simulink model "retail_store"  (R2014a)
settings: Solver=ode3  SolverMode=SingleTasking  StartTime=0.0  StopTime=24*3600  FixedStep=1  RelTol=1e-3
libraries: refrigeration x8
settings Model: Creator=avenger  LastModifiedBy=avenger
settings SolverCC: AutoInsertRateTranBlk=on
settings DataIOCC: LimitDataPoints=off
settings OptimizationCC: SimCompilerOptimization=off
settings DebuggingCC: MergeDetectMultiDrivingBlocksExec=error  FrameProcessingCompatibilityMsg=error
settings RTWCC: RTWCompilerOptimization=off

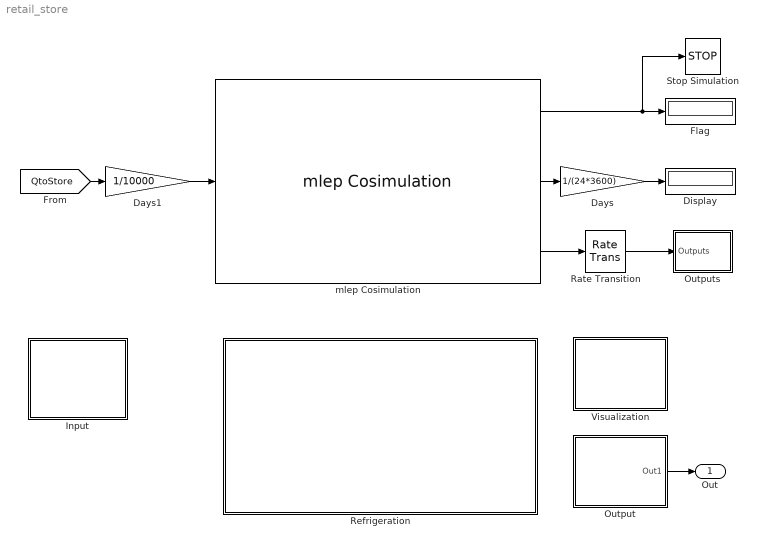
== system retail_store ==
  Days : Gain  Gain=1/(24*3600)
  Days1 : Gain  Gain=1/10000
  Display : Display
  Flag : Display
  Input : Subsystem
  Output : Subsystem
  Outputs : Subsystem
  Rate Transition : RateTransition
  Refrigeration : Subsystem
  Stop Simulation : Stop
  Visualization : Subsystem
  mlep Cosimulation : refrigeration/mlep Cosimulation  progname='runenergyplus'  idf='retail_810_cosim'  weather='USA_IL_Chicago-OHare.Intl.AP.725300_TMY3'  timeout=10000  step=300  numinput=1  numoutput=5  bcvtbpath='/home/ubuntu/mlep/bcvtb'
  Out : Outport  InitialOutput=0
  wires:
  mlep Cosimulation/2 -> Days/1
  mlep Cosimulation/1 -> Stop Simulation/1, Flag/1
  Days/1 -> Display/1
  mlep Cosimulation/3 -> Rate Transition/1
  [QtoStore] -> Days1/1
  Rate Transition/1 -> Outputs/1(Outputs)
  Days1/1 -> mlep Cosimulation/1
  Output/1(Out1) -> Out/1

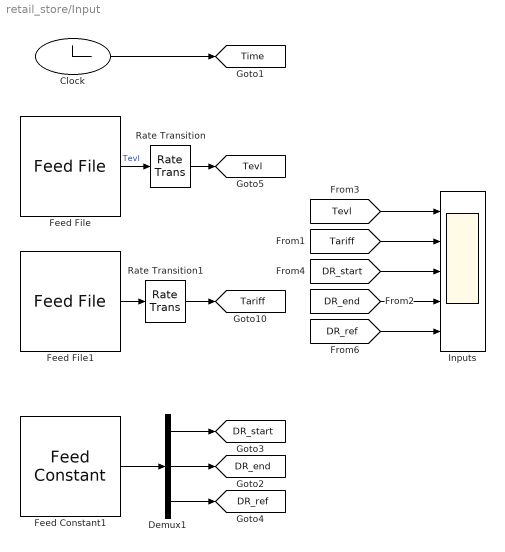
== system retail_store/Input ==
  Clock : Clock
  Demux1 : Demux  Outputs=3
  Feed Constant1 : refrigeration/Utilities/Feed Constant  filename='constant.txt'  timestep=300  numinput=3
  Feed File : refrigeration/Utilities/Feed File  filename='input.txt'  timestep=300  feedstep=3600
  Feed File1 : refrigeration/Utilities/Feed File  filename='input.txt'  timestep=300  feedstep=3600
  Inputs : Scope  NumInputPorts=5
      settings: ShowLegends=on  TimeRange=90000  YMin=0~0.02~14~14~399999  YMax=25~0.1~16~16~400001  SaveName=ScopeData3  SampleInput=on
  Rate Transition : RateTransition
  Rate Transition1 : RateTransition
  tag scope: DR_end=global, DR_ref=global, DR_start=global, Tariff=global, Tevl=global, Time=global
  wires:
  Feed File/1 -> Rate Transition/1  "Tevl"
  Clock/1 -> [Time]
  Feed File1/1 -> Rate Transition1/1
  Feed Constant1/1 -> Demux1/1
  [Tevl] -> Inputs/1
  [Tariff] -> Inputs/2
  Demux1/1 -> [DR_start]
  Demux1/2 -> [DR_end]
  Demux1/3 -> [DR_ref]
  [DR_start] -> Inputs/3
  [DR_end] -> Inputs/4
  [DR_ref] -> Inputs/5
  Rate Transition/1 -> [Tevl]
  Rate Transition1/1 -> [Tariff]

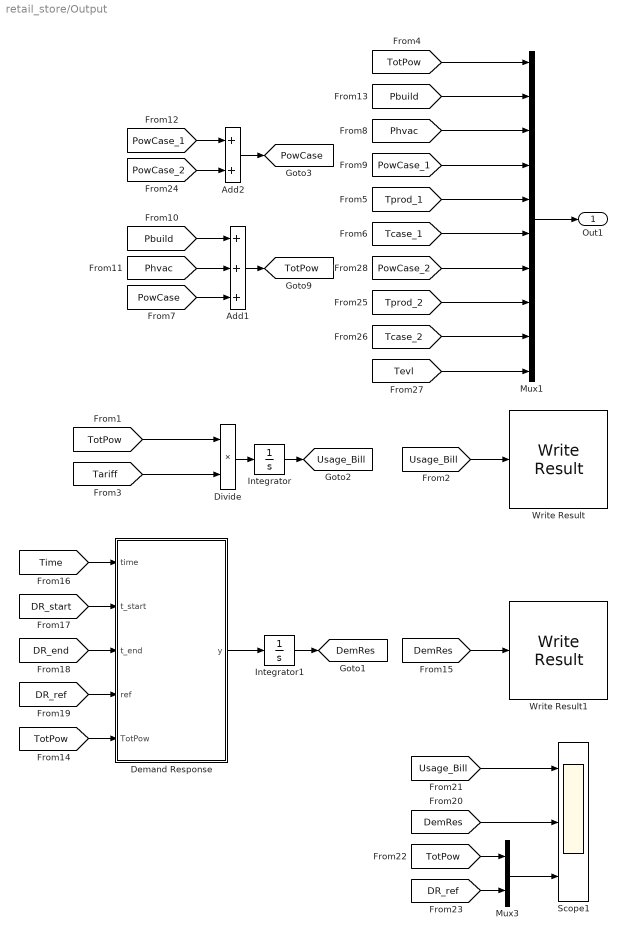
== system retail_store/Output ==
  Add1 : Sum  Inputs=+++
  Add2 : Sum
  Demand Response : MATLAB Function  TreatAsAtomicUnit=on
  Divide : Product  Inputs=**
  Integrator : Integrator  UpperSaturationLimit=10^7  LowerSaturationLimit=-10^7
  Integrator1 : Integrator  UpperSaturationLimit=10^7  LowerSaturationLimit=-10^7
  Mux1 : Mux  Inputs=10
  Mux3 : Mux  Inputs=2
  Scope1 : Scope  NumInputPorts=3
      settings: ShowLegends=on  TimeRange=90000  YMin=-200000000~0~-100000  YMax=1200000000~1200000000~500000  SaveName=ScopeData5
  Write Result : refrigeration/Utilities/Write Result  filename='result1.txt'  timestep=3600
  Write Result1 : refrigeration/Utilities/Write Result  filename='result2.txt'  timestep=3600
  Out1 : Outport  InitialOutput=0
  tag scope: DemRes=global, PowCase=global, TotPow=global, Usage_Bill=global
  wires:
  [Tariff] -> Divide/2
  Divide/1 -> Integrator/1
  [Pbuild] -> Add1/1
  [Phvac] -> Add1/2
  Add1/1 -> [TotPow]
  [Pbuild] -> Mux1/2
  [Tcase_1] -> Mux1/6
  [Tprod_1] -> Mux1/5
  [Phvac] -> Mux1/3
  [PowCase_1] -> Mux1/4
  [TotPow] -> Mux1/1
  Mux1/1 -> Out1/1
  Integrator/1 -> [Usage_Bill]
  [Usage_Bill] -> Write Result/1
  [DemRes] -> Write Result1/1
  [Time] -> Demand Response/1(time)
  [DR_start] -> Demand Response/2(t_start)
  [DR_end] -> Demand Response/3(t_end)
  [DR_ref] -> Demand Response/4(ref)
  [TotPow] -> Demand Response/5(TotPow)
  Demand Response/1(y) -> Integrator1/1
  Integrator1/1 -> [DemRes]
  [DemRes] -> Scope1/2
  [Usage_Bill] -> Scope1/1
  Mux3/1 -> Scope1/3
  [TotPow] -> Mux3/1
  [DR_ref] -> Mux3/2
  [TotPow] -> Divide/1
  [Tcase_2] -> Mux1/9
  [Tprod_2] -> Mux1/8
  [Tevl] -> Mux1/10
  [PowCase_2] -> Mux1/7
  [PowCase_1] -> Add2/1
  [PowCase_2] -> Add2/2
  Add2/1 -> [PowCase]
  [PowCase] -> Add1/3

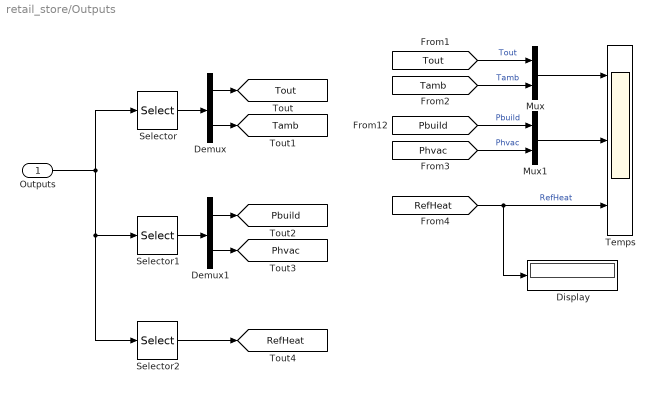
== system retail_store/Outputs ==
  Outputs : Inport
  Demux : Demux  Outputs=2
  Demux1 : Demux  Outputs=2
  Display : Display
  Mux : Mux  Inputs=2
  Mux1 : Mux  Inputs=2
  Selector : Selector  InputPortWidth=5  Indices=[1:2]
  Selector1 : Selector  InputPortWidth=5  Indices=[3:4]
  Selector2 : Selector  InputPortWidth=5  Indices=[5]
  Temps : Scope  NumInputPorts=3
      settings: ShowLegends=on  TimeRange=86400  YMin=0~0~-8000  YMax=32.5~375000~0
  tag scope: Pbuild=global, Phvac=global, RefHeat=global, Tamb=global, Tout=global
  wires:
  [Tout] -> Mux/1  "Tout"
  [Tamb] -> Mux/2  "Tamb"
  Mux/1 -> Temps/1
  [Pbuild] -> Mux1/1  "Pbuild"
  Selector/1 -> Demux/1
  Demux/1 -> [Tout]
  Demux/2 -> [Tamb]
  Selector1/1 -> Demux1/1
  Demux1/1 -> [Pbuild]
  Demux1/2 -> [Phvac]
  Mux1/1 -> Temps/2
  [Phvac] -> Mux1/2  "Phvac"
  Outputs/1 -> Selector2/1, Selector1/1, Selector/1
  Selector2/1 -> [RefHeat]
  [RefHeat] -> Display/1, Temps/3  "RefHeat"

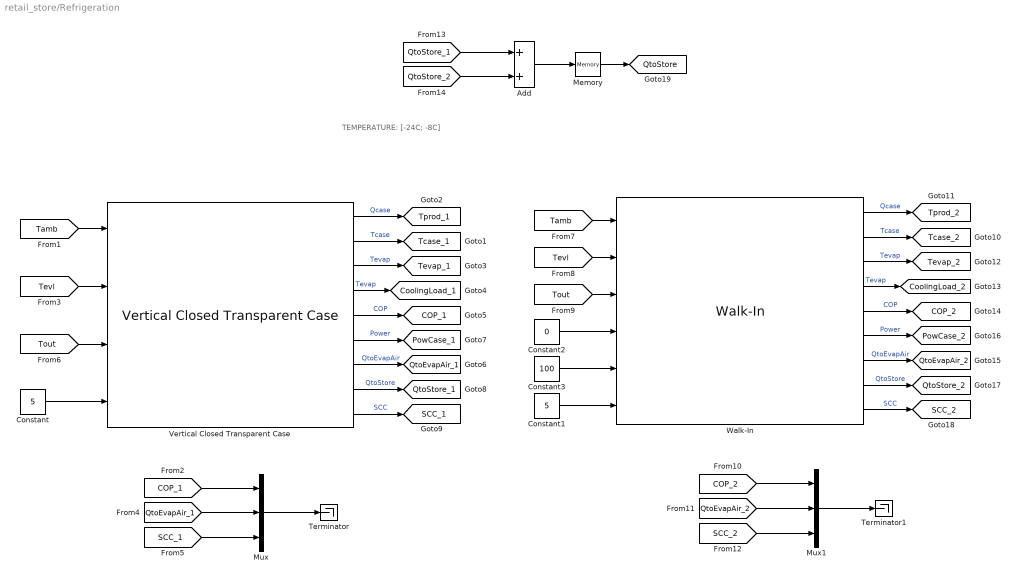
== system retail_store/Refrigeration ==
  note: TEMPERATURE: [-24C; -8C]
  Add : Sum
  Constant : Constant  Value=5
  Constant1 : Constant  Value=5
  Constant2 : Constant  Value=0
  Constant3 : Constant  Value=100
  Memory : Memory  X0=10000
  Mux : Mux  Inputs=3
  Mux1 : Mux  Inputs=3
  Terminator : Terminator
  Terminator1 : Terminator
  Vertical Closed Transparent Case : refrigeration/Refrigeration/Vertical Closed Transparent Case  Tcase_0=-12  Tprod_0=-12  Tevap_0=-12  Cprod=9.6310e4  Rcase=7.7559e-2  Ccase=9.4247e5  Beta=1.0376e-2  Alpha=3.8101e-2  Gamma=1.2792e-2  RatedLoad=4255  Qinternal=1484  LHR=0.1011  Cevap=150000  p_value=500
  Walk-In : refrigeration/Refrigeration/Walk-In  Tcase_0=-12  Tprod_0=-12  Tevap_0=-12  Cprod=9.6353e4  Rcase=9.6362e-2  Ccase=9.9033e5  Alpha=3.3139e-2  RatedLoad=4255  Qfan=329  Qlights=62  LHR=0  Cevap=400000  p_value=400
  tag scope: COP_1=global, COP_2=global, CoolingLoad_1=global, CoolingLoad_2=global, PowCase_1=global, PowCase_2=global, QtoEvapAir_1=global, QtoEvapAir_2=global, QtoStore=global, QtoStore_1=global, QtoStore_2=global, SCC_1=global, SCC_2=global, Tcase_1=global, Tcase_2=global, Tevap_1=global, Tevap_2=global, Tprod_1=global, Tprod_2=global
  wires:
  [Tevl] -> Vertical Closed Transparent Case/2
  Constant/1 -> Vertical Closed Transparent Case/4
  [Tamb] -> Vertical Closed Transparent Case/1
  [Tout] -> Vertical Closed Transparent Case/3
  Vertical Closed Transparent Case/1 -> [Tprod_1]  "Qcase"
  Vertical Closed Transparent Case/2 -> [Tcase_1]  "Tcase"
  Vertical Closed Transparent Case/3 -> [Tevap_1]  "Tevap"
  Vertical Closed Transparent Case/6 -> [PowCase_1]  "Power"
  Vertical Closed Transparent Case/8 -> [QtoStore_1]  "QtoStore"
  Vertical Closed Transparent Case/4 -> [CoolingLoad_1]  "Tevap"
  Vertical Closed Transparent Case/5 -> [COP_1]  "COP"
  Vertical Closed Transparent Case/7 -> [QtoEvapAir_1]  "QtoEvapAir"
  Vertical Closed Transparent Case/9 -> [SCC_1]  "SCC"
  [Tevl] -> Walk-In/2
  Constant1/1 -> Walk-In/6
  [Tamb] -> Walk-In/1
  [Tout] -> Walk-In/3
  Constant2/1 -> Walk-In/4
  Constant3/1 -> Walk-In/5
  Walk-In/1 -> [Tprod_2]  "Qcase"
  Walk-In/2 -> [Tcase_2]  "Tcase"
  Walk-In/3 -> [Tevap_2]  "Tevap"
  Walk-In/6 -> [PowCase_2]  "Power"
  Walk-In/8 -> [QtoStore_2]  "QtoStore"
  Walk-In/4 -> [CoolingLoad_2]  "Tevap"
  Walk-In/5 -> [COP_2]  "COP"
  Walk-In/7 -> [QtoEvapAir_2]  "QtoEvapAir"
  Walk-In/9 -> [SCC_2]  "SCC"
  [QtoEvapAir_1] -> Mux/2
  [SCC_1] -> Mux/3
  [COP_1] -> Mux/1
  Mux/1 -> Terminator/1
  [QtoEvapAir_2] -> Mux1/2
  [SCC_2] -> Mux1/3
  [COP_2] -> Mux1/1
  Mux1/1 -> Terminator1/1
  [QtoStore_2] -> Add/2
  [QtoStore_1] -> Add/1
  Memory/1 -> [QtoStore]
  Add/1 -> Memory/1

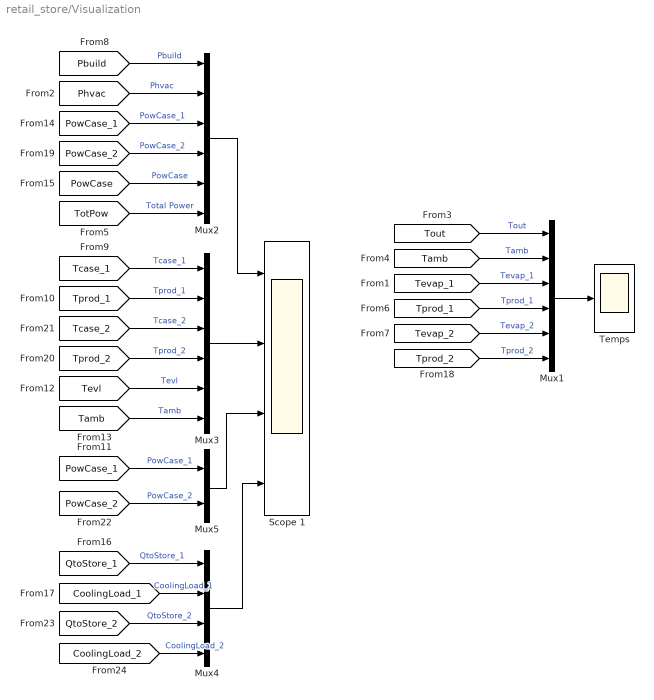
== system retail_store/Visualization ==
  Mux1 : Mux  Inputs=6
  Mux2 : Mux  Inputs=6
  Mux3 : Mux  Inputs=6
  Mux4 : Mux
  Mux5 : Mux  Inputs=2
  Scope 1 : Scope  NumInputPorts=4
      settings: ShowLegends=on  TimeRange=90000  YMin=0~-30~6000~-10000  YMax=100000~30~14000~30000  SaveName=ScopeData4
  Temps : Scope
      settings: ShowLegends=on  TimeRange=90000  YMin=0  YMax=35
  wires:
  Mux1/1 -> Temps/1
  [Tout] -> Mux1/1  "Tout"
  [Tamb] -> Mux1/2  "Tamb"
  [Tevap_1] -> Mux1/3  "Tevap_1"
  [Tprod_1] -> Mux1/4  "Tprod_1"
  [Pbuild] -> Mux2/1  "Pbuild"
  [Tcase_1] -> Mux3/1  "Tcase_1"
  [Tprod_1] -> Mux3/2  "Tprod_1"
  [Tevl] -> Mux3/5  "Tevl"
  [Tamb] -> Mux3/6  "Tamb"
  [PowCase_1] -> Mux2/3  "PowCase_1"
  Mux2/1 -> Scope 1/1
  [PowCase_1] -> Mux5/1  "PowCase_1"
  Mux3/1 -> Scope 1/2
  [Phvac] -> Mux2/2  "Phvac"
  [TotPow] -> Mux2/6  "Total Power"
  [QtoStore_1] -> Mux4/1  "QtoStore_1"
  [CoolingLoad_1] -> Mux4/2  "CoolingLoad_1"
  Mux4/1 -> Scope 1/4
  [Tevap_2] -> Mux1/5  "Tevap_2"
  [Tprod_2] -> Mux1/6  "Tprod_2"
  [PowCase_2] -> Mux2/4  "PowCase_2"
  [Tcase_2] -> Mux3/3  "Tcase_2"
  [Tprod_2] -> Mux3/4  "Tprod_2"
  [PowCase_2] -> Mux5/2  "PowCase_2"
  Mux5/1 -> Scope 1/3
  [QtoStore_2] -> Mux4/3  "QtoStore_2"
  [CoolingLoad_2] -> Mux4/4  "CoolingLoad_2"
  [PowCase] -> Mux2/5  "PowCase"

== matlab function retail_store/Output/MATLAB Function ==
  data: time input; y output; t_start input; t_end input; ref input; TotPow input
function y = fcn(time,t_start,t_end,ref,TotPow)
%#codegen


if (time > t_start*3600 && time < t_end*3600)
    y = TotPow - ref;
else
    y = 0;
end

== matlab function retail_store/Output/Demand Response ==
  data: time input; y output; t_start input; t_end input; ref input; TotPow input
function y = fcn(time,t_start,t_end,ref,TotPow)
%#codegen
 
if (time > t_start*3600 && time < t_end*3600)
    y = TotPow - ref;
else
    y = 0;
end
